simulink model "modelZSBwyy"  (Simulink 8.3)
settings: Solver=ode4  StartTime=0.0  StopTime=2  FixedStep=0.0001  RelTol=1e-3
settings Model: Creator=Chan Hwaiwing  LastModifiedBy=shubo
settings DataIOCC: LimitDataPoints=off  SignalLoggingSaveFormat=Dataset
settings OptimizationCC: OptimizeModelRefInitCode=on  LifeSpan=1
settings DebuggingCC: UnderspecifiedInitializationDetection=Simplified  MergeDetectMultiDrivingBlocksExec=error  FrameProcessingCompatibilityMsg=error  StateNameClashWarn=none
settings RTWCC: SystemTargetFile=ert.tlc  GenCodeOnly=on  PackageGeneratedCodeAndArtifacts=on  PackageName=zhusaibeng  TemplateMakefile=ert_default_tmf  Description=Embedded Coder  ProcessScript=ert_make_rtw_hook  BuildConfiguration=Faster Runs  TargetLang=C++
settings ERTTargetCC: MultiwordLength=2048  GenerateSampleERTMain=on  MultiInstanceERTCode=on  CodeInterfacePackaging=C++ class  SupportContinuousTime=on  RootIOFormat=Structure reference  ERTCustomFileTemplate=example_file_process.tlc  ConvertIfToSwitch=off  SuppressUnreachableDefaultCases=off
settings CPPComponent: GenerateDestructor=on  GenerateExternalIOAccessMethods=None  ParameterMemberVisibility=private  InternalMemberVisibility=private  GenerateParameterAccessMethods=None  GenerateInternalMemberAccessMethods=None  UseOperatorNewForModelRefRegistration=off

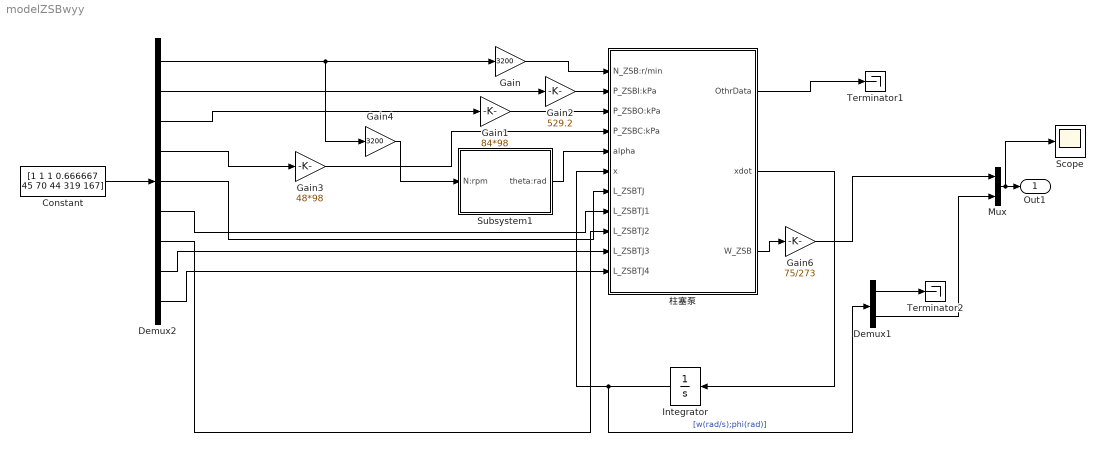
== system modelZSBwyy ==
  Constant : Constant  Value=[1 1 1 0.666667 45 70 44 319 167]
  Demux1 : Demux  Outputs=2
  Demux2 : Demux  Outputs=9
  Gain : Gain  Gain=3200
  Gain1 : Gain  Gain=84*98
  Gain2 : Gain  Gain=529.2
  Gain3 : Gain  Gain=48*98
  Gain4 : Gain  Gain=3200
  Gain6 : Gain  Gain=75/273
  Integrator : Integrator  InitialCondition=0.0001/180*pi  LimitOutput=on  UpperSaturationLimit=[inf 14.8/180*pi]  LowerSaturationLimit=[-inf 0]
  Mux : Mux  Inputs=2
  Scope : Scope
  Subsystem1 : Subsystem
  Terminator1 : Terminator
  Terminator2 : Terminator
  柱塞泵 : Subsystem  mask(柱塞泵){L_ZSBHX=15, D_ZSBZS=48*2, A_ZSBZS=23.8*23.8*pi/4, RHO=780, ETA_V=0.95, Z_ZSBZS=7, BETA_ZSBZS=12/180*pi, A_ZSBTJ=[pi*(33.26^2-17^2)/4, pi*(33.26^2-19.8^2)/4], k=((1421-754.6)/((139.7-101.9)-(139.7-119.6))+(1754-1313)/((158-96.8)-(158-114.6)))*1e3, BETA_ZSBSD=6.97/180*pi, L_x0=29.95+139.7, J_ZSBXP=0.34, KD=7.65}
      mask prompts: L_ZSBHX "L_ZSBHX(等效滑靴厚度mm)"; D_ZSBZS "D_ZSBZS(柱塞轴线在缸体的分布圆直径mm)"; A_ZSBZS "A_ZSBZS(柱塞截面面积mm^2)"; RHO "RHO(标准状态下，油液密度kg/m^3)"; ETA_V "ETA_V(容积效率)"; Z_ZSBZS "Z_ZSBZS(柱塞数量)"; BETA_ZSBZS "BETA_ZSBZS(柱塞安装角rad)"; A_ZSBTJ "A_ZSBTJ(面积参数向量mm^2)"; k "k(弹簧弹性模量N/m)"; BETA_ZSBSD "BETA_ZSBSD(随动活塞安装角rad)"; L_x0 "L_x0(随动活塞初始位置mm)"; J_ZSBXP "J_ZSBXP(斜盘绕斜盘轴的转动惯量kg·m^2)"; KD "KD(斜盘转动阻力系数N·m·s/rad)"
      mask DialogControl DescTextVar Prompt: 填入相关参数
  Out1 : Outport
  wires:
  Integrator/1 -> Demux1/1, 柱塞泵/6(x)  "[w(rad/s);phi(rad)]"
  Subsystem1/1(theta:rad) -> 柱塞泵/5(alpha)
  柱塞泵/2(xdot) -> Integrator/1
  柱塞泵/1(OthrData) -> Terminator1/1
  Demux2/4 -> Gain3/1
  Demux2/2 -> Gain2/1
  Demux2/3 -> Gain1/1
  Demux2/1 -> Gain4/1, Gain/1
  Mux/1 -> Scope/1, Out1/1
  Constant/1 -> Demux2/1
  Gain/1 -> 柱塞泵/1(N_ZSB:r/min)
  Gain2/1 -> 柱塞泵/2(P_ZSBI:kPa)
  Gain1/1 -> 柱塞泵/3(P_ZSBO:kPa)
  Gain3/1 -> 柱塞泵/4(P_ZSBC:kPa)
  Gain4/1 -> Subsystem1/1(N:rpm)
  柱塞泵/3(W_ZSB) -> Gain6/1
  Demux1/2 -> Mux/2
  Demux1/1 -> Terminator2/1
  Gain6/1 -> Mux/1
  Demux2/5 -> 柱塞泵/7(L_ZSBTJ)
  Demux2/6 -> 柱塞泵/8(L_ZSBTJ1)
  Demux2/7 -> 柱塞泵/9(L_ZSBTJ2)
  Demux2/8 -> 柱塞泵/10(L_ZSBTJ3)
  Demux2/9 -> 柱塞泵/11(L_ZSBTJ4)

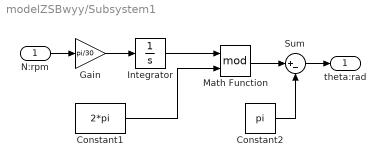
== system modelZSBwyy/Subsystem1 ==
  N:rpm : Inport
  Constant1 : Constant  Value=2*pi
  Constant2 : Constant  Value=pi
  Gain : Gain  Gain=pi/30
  Integrator : Integrator
  Math Function : Math  Operator=mod  SaturateOnIntegerOverflow=on
  Sum : Sum  Inputs=|+-
  theta:rad : Outport
  wires:
  Math Function/1 -> Sum/1
  N:rpm/1 -> Gain/1
  Constant1/1 -> Math Function/2
  Integrator/1 -> Math Function/1
  Gain/1 -> Integrator/1
  Sum/1 -> theta:rad/1
  Constant2/1 -> Sum/2

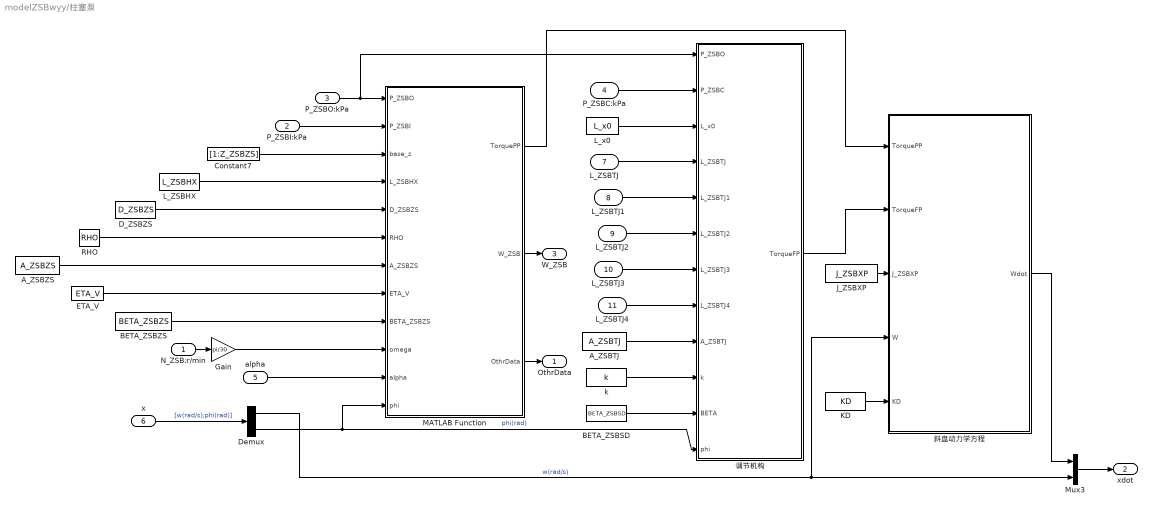
== system modelZSBwyy/柱塞泵 ==
  N_ZSB:r/min : Inport
  P_ZSBI:kPa : Inport  Port=2
  P_ZSBO:kPa : Inport  Port=3
  P_ZSBC:kPa : Inport  Port=4
  alpha : Inport  Port=5
  x : Inport  Port=6
  L_ZSBTJ : Inport  Port=7
  L_ZSBTJ1 : Inport  Port=8
  L_ZSBTJ2 : Inport  Port=9
  L_ZSBTJ3 : Inport  Port=10
  L_ZSBTJ4 : Inport  Port=11
  A_ZSBTJ : Constant  Value=A_ZSBTJ
  A_ZSBZS : Constant  Value=A_ZSBZS
  BETA_ZSBSD : Constant  Value=BETA_ZSBSD
  BETA_ZSBZS : Constant  Value=BETA_ZSBZS
  Constant7 : Constant  Value=[1:Z_ZSBZS]
  D_ZSBZS : Constant  Value=D_ZSBZS
  Demux : Demux  Outputs=2
  ETA_V : Constant  Value=ETA_V
  Gain : Gain  Gain=pi/30
  J_ZSBXP : Constant  Value=J_ZSBXP
  KD : Constant  Value=KD
  L_ZSBHX : Constant  Value=L_ZSBHX
  L_x0 : Constant  Value=L_x0
  MATLAB Function : MATLAB Function  TreatAsAtomicUnit=on
  Mux3 : Mux  Inputs=2
  RHO : Constant  Value=RHO
  k : Constant  Value=k
  斜盘动力学方程 : MATLAB Function  TreatAsAtomicUnit=on
  调节机构 : MATLAB Function  TreatAsAtomicUnit=on
  OthrData : Outport
  xdot : Outport  Port=2
  W_ZSB : Outport  Port=3
  wires:
  x/1 -> Demux/1  "[w(rad/s);phi(rad)]"
  斜盘动力学方程/1(Wdot) -> Mux3/1
  Mux3/1 -> xdot/1
  MATLAB Function/3(OthrData) -> OthrData/1
  alpha/1 -> MATLAB Function/11(alpha)
  J_ZSBXP/1 -> 斜盘动力学方程/3(J_ZSBXP)
  A_ZSBTJ/1 -> 调节机构/9(A_ZSBTJ)
  BETA_ZSBZS/1 -> MATLAB Function/9(BETA_ZSBZS)
  D_ZSBZS/1 -> MATLAB Function/5(D_ZSBZS)
  Demux/1 -> 斜盘动力学方程/4(W), Mux3/2  "w(rad/s)"
  k/1 -> 调节机构/10(k)
  L_x0/1 -> 调节机构/3(L_x0)
  Gain/1 -> MATLAB Function/10(omega)
  BETA_ZSBSD/1 -> 调节机构/11(BETA)
  P_ZSBO:kPa/1 -> 调节机构/1(P_ZSBO), MATLAB Function/1(P_ZSBO)
  L_ZSBTJ/1 -> 调节机构/4(L_ZSBTJ)
  L_ZSBHX/1 -> MATLAB Function/4(L_ZSBHX)
  RHO/1 -> MATLAB Function/6(RHO)
  Constant7/1 -> MATLAB Function/3(base_z)
  N_ZSB:r/min/1 -> Gain/1
  Demux/2 -> MATLAB Function/12(phi), 调节机构/12(phi)  "phi(rad)"
  P_ZSBC:kPa/1 -> 调节机构/2(P_ZSBC)
  P_ZSBI:kPa/1 -> MATLAB Function/2(P_ZSBI)
  调节机构/1(TorqueFP) -> 斜盘动力学方程/2(TorqueFP)
  KD/1 -> 斜盘动力学方程/5(KD)
  MATLAB Function/1(TorquePP) -> 斜盘动力学方程/1(TorquePP)
  A_ZSBZS/1 -> MATLAB Function/7(A_ZSBZS)
  ETA_V/1 -> MATLAB Function/8(ETA_V)
  MATLAB Function/2(W_ZSB) -> W_ZSB/1
  L_ZSBTJ1/1 -> 调节机构/5(L_ZSBTJ1)
  L_ZSBTJ2/1 -> 调节机构/6(L_ZSBTJ2)
  L_ZSBTJ4/1 -> 调节机构/8(L_ZSBTJ4)
  L_ZSBTJ3/1 -> 调节机构/7(L_ZSBTJ3)

== matlab function 柱塞泵/MATLAB Function ==
  data: P_ZSBO input double; TorquePP output double; P_ZSBI input double; base_z input double; L_ZSBHX input double; D_ZSBZS input double; RHO input double; A_ZSBZS input double; ETA_V input double; BETA_ZSBZS input double; omega input double; alpha input double; phi input double; W_ZSB output double; OthrData output double
% function [ TorquePP,W_ZSB,OthrData ] = Plunger_Pump(P_ZSBO,  P_ZSBI,  base_z, L_ZSBHX, D_ZSBZS, RHO, A_ZSBZS, ETA_V,BETA_ZSBZS,omega,alpha,phi )
% CF = 1.00;
% %% ****** Plunger Centroid Calculate BEGIN *****
% dz = (23.7820+23.8074+23.8328+23.8582+23.8836)*CF/5;
% d11 = 22.6*CF;
% d12 = 19*CF;
% l1 = 2.9*CF;
% V1a = pi/3*l1*(d11*d11/4+d12*d12/4+d11*d12/4);
% V1b = pi/4*dz*dz*l1;
% V1 = V1b-V1a;
% lr = 48.8*CF;
% l2 = lr-l1;
% d2 = 19*CF;
% V2 = pi/4*(dz*dz-d2*d2)*l2;
% l3 = (5.5-3.2)/2/tan(60*pi/180)*CF;
% d31 = 5.5*CF;
% d32 = 3.2*CF;
% V3a = pi/3*l3*(d31*d31/4+d32*d32/4+d31*d32/4);
% V3b = pi/4*dz*dz*l3;
% V3 = V3b-V3a;
% l4 = (51.5-48.8)*CF-l3;
% d4 = 3.2*CF;
% V4 = pi/4*(dz*dz-d4*d4)*l4;
% l5 = 5/2*sin(45*pi/180)*CF;
% d51 = dz;
% d52 = dz-2*5/2*cos(45*pi/180)*CF;
% d5 = 3.2*CF;
% V5a = pi/4*d5*d5*l5;
% V5b = pi/3*l5*(d51*d51/4+d52*d52/4+d51*d52/4);
% V5 = V5b-V5a;
% l6 = 7.4/2*sin(20*pi/180)*CF;
% d61 = d52;
% d62 = 12.8*CF;
% d6 = 3.2*CF;
% V6a = pi/4*d6*d6*l6;
% V6b =  pi/3*l6*(d61*d61/4+d62*d62/4+d61*d62/4);
% V6 = V6b-V6a;
% l7 = (17.2-16)*CF;
% d71 = 12.8*CF;
% d72 = 3.2*CF;
% V7 = pi/4*(d71*d71-d72*d72)*l7;
% SR = 19.05/2*CF;
% d8 = 3.2*CF;
% d81 = 12.8*CF;
% d82 = 5*CF;
% l81 = SR-sqrt(SR*SR-d81*d81/4);
% l82 = SR-sqrt(SR*SR-d82*d82/4);
% l8 = 2*SR - l81 - l82;
% V81 = pi/3*l81*l81*(3*SR-l81);
% V82 = pi/3*l82*l82*(3*SR-l82);
% VS8 = 4/3*pi*SR*SR*SR;
% V83 = pi/4*d8*d8*l8;
% V8 = VS8-V81-V82-V83;
% X1a = l1*(d11*d11/4+2*d11/2*d12/2+3*d12*d12/4)/4/(d11*d11/4+d11/2*d12/2+d12*d12/4);
% X1b = l1/2;
% X1 = (V1b*X1b-V1a*X1a)/(V1b-V1a);
% X2p = l2/2;
% X2 = X2p+l1;
% X3a = l3*(d31*d31/4+2*d31/2*d32/2+3*d32*d32/4)/4/(d31*d31/4+d31/2*d32/2+d32*d32/4);
% X3b = l3/2;
% X3p = (V3b*X3b-V3a*X3a)/(V3b-V3a);
% X3 = X3p+lr;
% X4p = l4/2;
% X4 = X4p+48.8*CF+l3;
% X5a = l5/2;
% X5b = l5*(d51*d51/4+2*d51/2*d52/2+3*d52*d52/4)/4/(d51*d51/4+d51/2*d52/2+d52*d52/4);
% X5p = (V5b*X5b-V5a*X5a)/(V5b-V5a);
% X5 = X5p+51.5*CF;
% X6a = l6/2;
% X6b = l6*(d61*d61/4+2*d61/2*d62/2+3*d62*d62/4)/4/(d61*d61/4+d61/2*d62/2+d62*d62/4);
% X6p = (V6b*X6b-V6a*X6a)/(V6b-V6a);
% X6 = X6p+51.5*CF+l5;
% X7p = l7/2;
% X7 = X7p+51.5*CF+l5+l6;
% X8a = SR-3*(2*SR-l81)*(2*SR-l81)/4/(3*SR-l81);
% X8b = SR+3*(2*SR-l82)*(2*SR-l82)/4/(3*SR-l82);
% X8c = SR;
% X8d = (VS8*X8c-V81*X8a-V82*X8b)/(VS8-V81-V82)-l81;
% X8e = l8/2;
% X8p = ((VS8-V81-V82)*X8d - V83*X8e)/(VS8-V81-V82-V83);
% X8 = X8p+(72.62-16)*CF;
% Xc = (V1*X1+V2*X2+V3*X3+V4*X4+V5*X5+V6*X6+V7*X7+V8*X8)/(V1+V2+V3+V4+V5+V6+V7+V8);
% k=63.2*CF-Xc;
% mz=0.1006*CF;
% %% ****** Plunger Centroid Calculate END *********
% %% ****** Plunger Kinematics Calculate BEGIN *****
% R = 266.7*CF;
% theta = 11*pi/180;
% dz = (23.7820+23.8074+23.8328+23.8582+23.8836)*CF/5;
% h = 17*0.45/0.6*CF;
% etaV = 0.95;
% z = 7;
% a = R/cos(theta);
% c = a;
% R0 = sqrt(c*c+a*a-2*c*a*cos(phi));
% tau = atan((cos(phi)-a/c)/sin(phi));
% L = R-h;
% lambda = R0/L;
% A1 = -cos(theta)*sin(tau);
% B1 = -sin(theta)*cos(tau);
% D = 1+lambda*A1-lambda*lambda*(1-A1*A1-B1*B1/2)/2;
% E = lambda*B1*(1+lambda*A1);
% F = lambda*lambda*B1*B1;
% Smax = -2*L.*E;
% %% ****** Plunger Kinematics Calculate END *****
% %% ****** Plunger Force and total Torque Calculation BEGIN ******
% r1 = 35/2*CF;
% r2 = 57.8*CF*cos(15*pi/180);
% rou_fuel = 775;
% kesi = 0.75;
% Kt = (70.27-9.11)/((77.3-50.2)-(77.3-73.8));
% l01 = 77.3*CF;
% b = (82.55/2/sin(10*pi/180)-69)*CF;
% e1 = 7.2*CF;
% e2 = 2.5*CF;
% e3 = (63.2-48.8)*CF;
% r=D_ZSBZS/2;
% z = length( base_z );
% S_max = 2 * r * tan( phi );
% alpha_tab =  alpha + base_z * 2 * pi / z;
% v_tab = -r * sin( alpha_tab ) * tan( phi ) * omega;
% l_tab = r * cos( alpha_tab ) / cos( phi ) + L_ZSBHX * tan( phi );
% s1=2*r*tan(phi);
% acc = -L*omega*omega*(E*cos(alpha_tab)+F*cos(2*alpha_tab));
% v_tab1 = L*omega*(E*sin(alpha_tab)+F*sin(2*alpha_tab)/2);
% p_tab = base_z;
% R = 266.7;
% a = R/cos(BETA_ZSBZS);
% c = a;
% R0 = sqrt(c*c+a*a-2*c*a*cos(phi));
% h = 17*0.45/0.6;
% L = R-h;
% lambda = R0/L;
% tau = atan((cos(phi)-a/c)/sin(phi));
% A1 = -cos(BETA_ZSBZS)*sin(tau);
% B1 = -sin(BETA_ZSBZS)*cos(tau);
% D = 1+lambda*A1-lambda*lambda*(1-A1*A1-B1*B1/2)/2;
% E = lambda*B1*(1+lambda*A1);
% F = lambda*lambda*B1*B1;
% rou = L*(D+E*cos(alpha_tab)+F*cos(2*alpha_tab)/4);
% a5=rou.*rou;
% phi2 = acos((a5+L*L-R0*R0)/2./rou/L);
% for i = 1 : z
%     if ( alpha_tab( i ) >= pi )
%         alpha_tab( i ) =  alpha_tab( i ) - 2 * pi;
%     end
%     if ( alpha_tab( i ) < 0 )
%         p_tab( i ) = P_ZSBO;
%     else
%         p_tab( i ) = P_ZSBI;
%         v_tab( i ) = 0;
%         v_tab1(i)=0;
%     end
% end
% k=24.0668;
% mz=0.1006;
% dzr = 3.2;
% rou_fuel = 775;
% kesi = 0.75;
% r1 = 35/2;
% r2 = 57.8*cos(15*pi/180);
% d_yaotou = 17*1.0/0.6;
% dz = (23.7820+23.8074+23.8328+23.8582+23.8836)/5;
% FL=mz*omega*omega*(rou-k)*1e-3*sin(BETA_ZSBZS);%/N
% FLz=FL*sin(BETA_ZSBZS);
% Pz = P_ZSBI+rou_fuel/2*kesi*(r2*r2-r1*r1)*1e-6*omega*omega*1e-3;%--转子腔油压，/Mpa
% Fu2 = pi/4*(d_yaotou*d_yaotou-(dz*dz-dzr*dzr)*cos(phi2))*1e-6*Pz*1e3;%--fuel pressure force,/N
% % plunger spring force
% Ft = Kt*(b+e1+l01+e2+e3)-Kt*rou;%--spring force,/N
% % New Add Cage spring force
% l02 = 56.6;
% Kt2 = 44.39/(56.6-14.3);
% % washer thickness
% t2 = (1.05+1.10+1.20+1.30+1.35+1.40+1.55+1.60+1.65+1.80+1.95)/11;
% B2 = 19.7+t2+6.4-12.8;
% Ft2 = Kt2*(l02 - B2);
% Ft2f = Ft2/cos(phi);
% theta_f = 10*pi/180;
% Ft2i = Ft2f/cos(theta_f)/z;
% % plunger centrifugal force
% FL = mz*omega*omega*(rou-k)*1e-3*sin(theta);%/N
% FLz = FL*sin(theta);
% %FLy = FL*cos(theta);%--Centrifugal force+Ft2i
% % relative motion inertial force
% Fg = -mz*acc*1e-3;%--inertia force
% A11 = ((a+R0*sin(tau))*sin(BETA_ZSBZS)*cos(alpha_tab)-R0*cos(tau)*cos(BETA_ZSBZS))/L;%--total force, one piston, on plate
% h1 = a*R0*cos(tau)/L;
% lt = A11.*rou+h1;
% F1=A_ZSBZS * p_tab*1e-3;
% f_tab=(A_ZSBZS * p_tab+Fg*1e3+Ft*1e3+FLz*1e3)./cos( phi2)+(Fu2+Ft2i)*1e3;
% m_tab=l_tab.* f_tab * 1e-6;
% TorquePP=-sum( m_tab ); 
% %-- Calculate q_tab and total Q --
% q_tab = A_ZSBZS * ETA_V*cos(BETA_ZSBZS) * v_tab* RHO * 1e-9;
% W_ZSB = sum( q_tab );
% Q2 = RHO * ETA_V *cos(BETA_ZSBZS)* A_ZSBZS * S_max * z * omega * 0.5 / pi * 1e-9;
% OthrData = [ Q2, TorquePP, S_max, v_tab( z ), q_tab( z ), l_tab( z ), f_tab( z ), m_tab( z ) ];
% end
function [ TorquePP,W_ZSB,OthrData ] = Plunger_Pump(P_ZSBO,  P_ZSBI,  base_z, L_ZSBHX, D_ZSBZS, RHO, A_ZSBZS, ETA_V,BETA_ZSBZS,omega,alpha,phi )
r=D_ZSBZS/2;
z = length( base_z );
S_max = 2 * r * tan( phi );
alpha_tab =  alpha + base_z * 2 * pi / z;
v_tab = -r * sin( alpha_tab ) * tan( phi ) * omega;
l_tab = r * cos( alpha_tab ) / cos( phi ) + L_ZSBHX * tan( phi );
p_tab = base_z;
for i = 1 : z
    if ( alpha_tab( i ) >= pi )
        alpha_tab( i ) =  alpha_tab( i ) - 2 * pi;
    end
    if ( alpha_tab( i ) < 0 )
        p_tab( i ) = P_ZSBO;
    else
        p_tab( i ) = P_ZSBI;
        v_tab( i ) = 0;
    end
end
f_tab = A_ZSBZS * p_tab / cos( phi );
m_tab = l_tab .* f_tab * 1e-6;
TorquePP = -sum( m_tab ); 
%-- Calculate q_tab and total Q --
q_tab=A_ZSBZS*ETA_V*cos(BETA_ZSBZS)*v_tab*RHO*1e-9; 
W_ZSB = sum(q_tab);
Q2=RHO*ETA_V*cos(BETA_ZSBZS)*A_ZSBZS*S_max*z*omega*0.5/pi*1e-9;
OthrData = [ Q2, TorquePP, S_max, v_tab( z ), q_tab( z ), l_tab( z ), f_tab( z ), m_tab( z ) ];
end

== matlab function 柱塞泵/调节机构 ==
  data: P_ZSBO input double; TorqueFP output double; P_ZSBC input double; L_x0 input double; L_ZSBTJ input double; L_ZSBTJ1 input double; L_ZSBTJ2 input double; L_ZSBTJ3 input double; L_ZSBTJ4 input double; A_ZSBTJ input double; k input double; BETA input double; phi input double
function TorqueFP=TJ(P_ZSBO,P_ZSBC,L_x0,L_ZSBTJ,L_ZSBTJ1,L_ZSBTJ2,L_ZSBTJ3,L_ZSBTJ4,A_ZSBTJ,k,BETA,phi)
%计算活塞位置
xp=L_ZSBTJ3+L_ZSBTJ*sin(phi+BETA)-L_ZSBTJ4-sqrt(abs(L_ZSBTJ2*L_ZSBTJ2-(L_ZSBTJ1-L_ZSBTJ*cos(phi+BETA))^2));
%计算随动活塞杆上的作用力
Pleft=P_ZSBO*1e3;%Pa
Pright=Pleft-P_ZSBC*1e3;%Pa
Fleft=Pleft*A_ZSBTJ(1)*1e-6;%N
Fright=Pright*A_ZSBTJ(2)*1e-6;%N
Fs=k*(L_x0-xp)*1e-3;
Fsui=Fs +Fright-Fleft;
%计算随动活塞杆力对斜盘作用力矩
delta = asin((L_ZSBTJ1-L_ZSBTJ*cos(phi+BETA))/L_ZSBTJ2);
TorqueFP = (Fsui/cos(delta)*cos(delta-phi-BETA)*L_ZSBTJ*1e-3);
end

== matlab function 柱塞泵/斜盘动力学方程 ==
  data: TorquePP input double; Wdot output double; TorqueFP input double; J_ZSBXP input double; W input double; KD input double
function Wdot=DL(TorquePP,TorqueFP,J_ZSBXP,W,KD) 
Torq_Net=TorquePP+TorqueFP-W* KD;
Wdot=Torq_Net/J_ZSBXP;
end
